simulink model "mpc555rt_candb"  (Simulink 6.0)
settings: Solver=FixedStepDiscrete  StartTime=0.0  StopTime=inf  RelTol=1e-3
PreLoadFcn:
  | RTWConfigurationCB('preloadfcn', bdroot);
libraries: canblocks x3, mpc555drivers x3, mpc555toucan x3
CloseFcn:
  | rtwprivate ssgencode ModelCloseRequest mpc555rt_candb
settings Model: Creator=The MathWorks Inc.  LastModifiedBy=batserve  ExtModeAutoUpdateStatusClock=off  ProdHWDeviceType=Motorola PowerPC
settings DataIOCC: SignalLoggingName=sigsOut
settings OptimizationCC: InlineParams=on  InlineInvariantSignals=off  OptimizeModelRefInitCode=on  LifeSpan=1
settings DebuggingCC: CheckExecutionContextPreStartOutputMsg=on  CheckExecutionContextRuntimeOutputMsg=on  SolverPrmCheckMsg=none
settings HardwareCC: ProdEndianess=BigEndian  ProdHWDeviceType=Motorola PowerPC
settings ModelReferenceCC: UpdateModelReferenceTargets=IfOutOfDate
settings RTWCC: SystemTargetFile=mpc555rt.tlc  TemplateMakefile=mpc555rt.tmf  Description=Embedded Target for Motorola MPC555 (real-time target)  ProcessScript=mpc555rt_make_rtw_hook
settings CodeAppCC: IgnoreCustomStorageClasses=off
settings STFCustomTargetCC: TargetFcnLib=ansi_tfl_tmw.mat  GenFloatMathFcnCalls=ANSI_C  ModelReferenceCompliant=off  CombineOutputUpdateFcns=on  ERTCustomFileBanners=on  SystemTargetFile=mpc555rt.tlc
settings ERTTargetCC: TargetFcnLib=ansi_tfl_tmw.mat  GenFloatMathFcnCalls=ANSI_C  ModelReferenceCompliant=off  SupportContinuousTime=on  SupportNonInlinedSFcns=on  RootIOFormat=Individual Arguments  ERTCustomFileTemplate=example_file_process.tlc  InitialValueSource=Model
settings CustomProperty: DataType=RTWOptions_EnumType__toolbox_rtw_targets_mpc555dk_mpc555dk_mpc555rt_MPC555_OPTIMIZATION_SWITCH  Value=speed
settings EnumStrPairs: String=speed

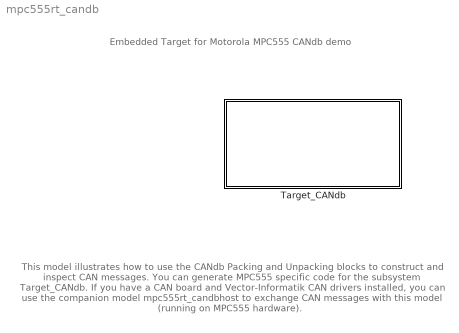
== system mpc555rt_candb ==
  note: Embedded Target for Motorola MPC555
      |                    CANdb demo
  note: This model illustrates how to use the CANdb Packing and Unpacking blocks
      | to construct and inspect CAN messages.
      |
      | You can generate MPC555 specific code for the subsystem Target_CANdb.
      |
      | If you have a CAN board and Vector-Informatik CAN drivers installed, you can use the
      | companion model mpc555rt_candbhost to exchange CAN messages with this model (running
      | on MPC555 hardware).
  Target_CANdb : Subsystem  InitFcn=|  PropExecContextAcrossSSBoundary=on
      | % START RTW CONFIGURATION CODE %
      | RTWConfigurationCB('rtw_target_initfcn',gcb);
      | % END RTW CONFIGURATION CODE %
      mask Display: image(imread('target_affordance_icon.jpg'),'bottom-right')

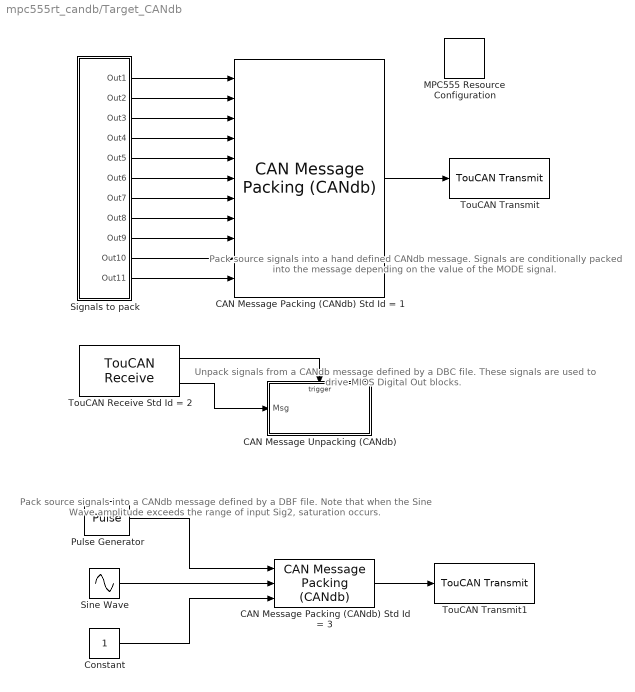
== system mpc555rt_candb/Target_CANdb ==
  note: Pack source signals into a hand
      | defined CANdb message. Signals
      | are conditionally packed into the
      | message depending on the value
      | of the MODE signal.
  note: Unpack signals from a CANdb message
      | defined by a DBC file.
      | These signals are used to drive MIOS
      | Digital Out blocks.
  note: Pack source signals into a CANdb message defined by a DBF file.
      | Note that when the Sine Wave amplitude exceeds the range of
      | input Sig2, saturation occurs.
  CAN Message Packing (CANdb) Std Id = 1 : canblocks/CAN Message Packing (CANdb)
  CAN Message Packing (CANdb) Std Id = 3 : canblocks/CAN Message Packing (CANdb)
  CAN Message Unpacking (CANdb) : Subsystem  TreatAsAtomicUnit=on  PropExecContextAcrossSSBoundary=on
  Constant : Constant
  MPC555 Resource Configuration : mpc555drivers/MPC555 Resource Configuration  Tag=RTW CONFIGURATION BLOCK  Priority=-100000  oldParentName=mpc555rt_candb/Target_CANdb  oldBlockName=|  defaultConfigLibrary=mpc555drivers
      | mpc555rt_candb/Target_CANdb/MPC555
      | Resource
      | Configuration
  Pulse Generator : DiscretePulseGenerator  SampleTime=0.1
  Signals to pack : Subsystem  PropExecContextAcrossSSBoundary=on
  Sine Wave : Sin  SineType=Sample based  Amplitude=70  Samples=50  SampleTime=0.1
  TouCAN Receive Std Id = 2 : mpc555toucan/TouCAN Receive  module=A  ids=2  notification_type=Function Call Outport  auto_select_buffer=on  bufferids=3  use_queue=off  queue_length=3  message_type=Standard (11-bit identifier)  t=0.1
  TouCAN Transmit : mpc555toucan/TouCAN Transmit  module=A  tx_mode=Queued transmission with shared buffer  fifo_queue_length=8  bufferids=0  t=-1  enablePassThru=off
  TouCAN Transmit1 : mpc555toucan/TouCAN Transmit  module=A  tx_mode=Queued transmission with shared buffer  fifo_queue_length=8  bufferids=0  t=-1  enablePassThru=off
  wires:
  CAN Message Packing (CANdb) Std Id = 3/1 -> TouCAN Transmit1/1
  Constant/1 -> CAN Message Packing (CANdb) Std Id = 3/3
  Sine Wave/1 -> CAN Message Packing (CANdb) Std Id = 3/2
  Pulse Generator/1 -> CAN Message Packing (CANdb) Std Id = 3/1
  CAN Message Packing (CANdb) Std Id = 1/1 -> TouCAN Transmit/1
  Signals to pack/11(Out11) -> CAN Message Packing (CANdb) Std Id = 1/11
  Signals to pack/10(Out10) -> CAN Message Packing (CANdb) Std Id = 1/10
  Signals to pack/9(Out9) -> CAN Message Packing (CANdb) Std Id = 1/9
  Signals to pack/8(Out8) -> CAN Message Packing (CANdb) Std Id = 1/8
  Signals to pack/7(Out7) -> CAN Message Packing (CANdb) Std Id = 1/7
  Signals to pack/6(Out6) -> CAN Message Packing (CANdb) Std Id = 1/6
  Signals to pack/5(Out5) -> CAN Message Packing (CANdb) Std Id = 1/5
  Signals to pack/4(Out4) -> CAN Message Packing (CANdb) Std Id = 1/4
  Signals to pack/3(Out3) -> CAN Message Packing (CANdb) Std Id = 1/3
  Signals to pack/2(Out2) -> CAN Message Packing (CANdb) Std Id = 1/2
  Signals to pack/1(Out1) -> CAN Message Packing (CANdb) Std Id = 1/1
  TouCAN Receive Std Id = 2/1 -> CAN Message Unpacking (CANdb)/Trigger
  TouCAN Receive Std Id = 2/2 -> CAN Message Unpacking (CANdb)/1(Msg)

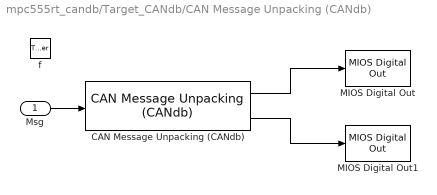
== system mpc555rt_candb/Target_CANdb/CAN Message Unpacking (CANdb) ==
  Msg : Inport  Port=1  LatchInput=off
  f : TriggerPort  TriggerType=function-call
  CAN Message Unpacking (CANdb) : canblocks/CAN Message Unpacking (CANdb)/CAN Message Unpacking (CANdb)
  MIOS Digital Out : mpc555drivers/Modular Input//Output System (MIOS1)/MIOS Digital Out  bits=0  init=0  t=-1  enablePassThru=off
  MIOS Digital Out1 : mpc555drivers/Modular Input//Output System (MIOS1)/MIOS Digital Out  bits=1  init=0  t=-1  enablePassThru=off
  wires:
  Msg/1 -> CAN Message Unpacking (CANdb)/1
  CAN Message Unpacking (CANdb)/1 -> MIOS Digital Out/1
  CAN Message Unpacking (CANdb)/2 -> MIOS Digital Out1/1

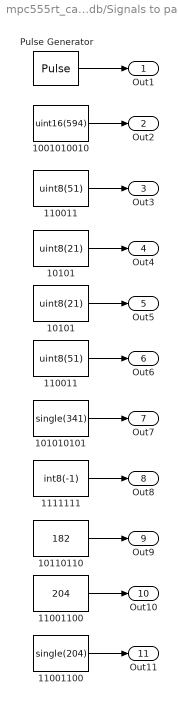
== system mpc555rt_candb/Target_CANdb/Signals to pack ==
  " 1001010010" : Constant  Value=uint16(594)
  " 10101 " : Constant  Value=uint8(21)
  " 101010101" : Constant  Value=single(341)
  " 110011 " : Constant  Value=uint8(51)
  " 11001100 " : Constant  Value=204
  10101 : Constant  Value=uint8(21)
  10110110 : Constant  Value=182
  110011 : Constant  Value=uint8(51)
  11001100 : Constant  Value=single(204)
  1111111 : Constant  Value=int8(-1)
  Pulse Generator : DiscretePulseGenerator  Period=100  PulseWidth=50  SampleTime=0.1
  Out1 : Outport
  Out2 : Outport  Port=2
  Out3 : Outport  Port=3
  Out4 : Outport  Port=4
  Out5 : Outport  Port=5
  Out6 : Outport  Port=6
  Out7 : Outport  Port=7
  Out8 : Outport  Port=8
  Out9 : Outport  Port=9
  Out10 : Outport  Port=10
  Out11 : Outport  Port=11
  wires:
  11001100/1 -> Out11/1
  " 11001100 "/1 -> Out10/1
  10110110/1 -> Out9/1
  1111111/1 -> Out8/1
  " 101010101"/1 -> Out7/1
  110011/1 -> Out6/1
  10101/1 -> Out5/1
  " 10101 "/1 -> Out4/1
  " 110011 "/1 -> Out3/1
  " 1001010010"/1 -> Out2/1
  Pulse Generator/1 -> Out1/1
